simulink model "Sensor_actuator_test"  (R2020b)
settings: Solver=FixedStepAuto  StartTime=0.0  StopTime=inf  FixedStep=1  RelTol=1e-7  EnableMultiTasking=on
libraries: embdlinuxlib x12
settings Model: SimulationMode=external  Creator=enzlp  LastModifiedBy=Triphase_Setup
settings SolverCC: AlgebraicLoopSolver=LineSearch  PositivePriorityOrder=on
settings DataIOCC: SaveFormat=Array  ReturnWorkspaceOutputs=off
settings OptimizationCC: EnhancedBackFolding=on  PassReuseOutputArgsAs=Individual arguments  ZeroExternalMemoryAtStartup=off  ZeroInternalMemoryAtStartup=off  MaxStackSize=64  OptimizeBlockOrder=speed  DifferentSizesBufferReuse=on  OptimizationCustomize=off  EfficientTunableParamExpr=on
settings DebuggingCC: ParameterTunabilityLossMsg=error
settings HardwareCC: ProdBitPerPointer=32  ProdBitPerSizeT=32  ProdBitPerPtrDiffT=32  ProdLargestAtomicInteger=Long  ProdLargestAtomicFloat=Double  ProdWordSize=32  ProdLongLongMode=on  ProdHWDeviceType=ARM Compatible->ARM Cortex
settings RTWCC: Description=Embedded Coder  SystemTargetFile=ert.tlc  HardwareBoard=Raspberry Pi  TLCOptions="-aInlineSetEventsForThisBaseRateFcn=TLC_FALSE -aSuppressMultiTaskScheduler=TLC_FALSE  -aRateBasedStepFcn=0"  TemplateMakefile=ert_default_tmf  Toolchain=GNU GCC Raspberry Pi  BuildConfiguration=Faster Runs
settings CodeAppCC: ForceParamTrailComments=on  IgnoreCustomStorageClasses=off  OperatorAnnotations=on  SimulinkDataObjDesc=on  SFDataObjDesc=on  InsertBlockDesc=on
settings ERTTargetCC: TargetLangStandard=C99 (ISO)  SupportVariableSizeSignals=on  ExtMode=on  ExtModeTransport=2  ExtModeStaticAlloc=on  ExtModeMexFile=ext_xcp  ExtModeMexArgs='192.168.178.34' 0 17725  ExtModeIntrfLevel=Level2 - Open

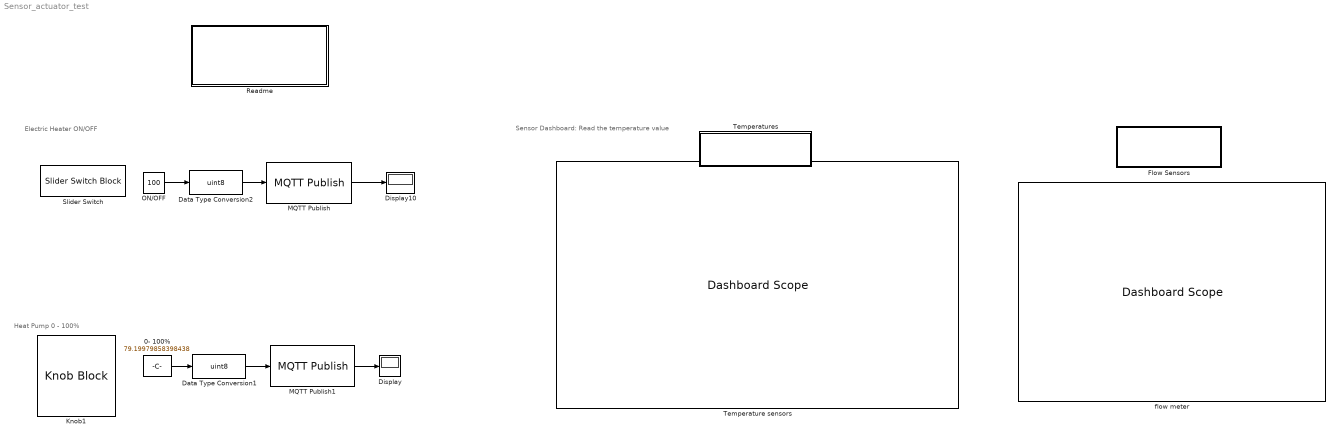
== system Sensor_actuator_test ==
  note: Heat Pump 0 - 100%
  note: Sensor Dashboard: Read the temperature value
  note: Electric Heater ON/OFF
  0- 100% : Constant  Value=79.19979858398438
  Data Type Conversion1 : DataTypeConversion  OutDataTypeStr=uint8
  Data Type Conversion2 : DataTypeConversion  OutDataTypeStr=uint8
  Display : Display
  Display10 : Display
  Flow Sensors : Subsystem
  Knob1 : KnobBlock
  MQTT Publish : embdlinuxlib/MQTT Publish  Topic=heatpump  QoS=0  RetainMsg=off
      settings: SourceProductBaseCode=SC_BEAGLEBONE_BLUE,NVIDIA,RASPPI
  MQTT Publish1 : embdlinuxlib/MQTT Publish  Topic=boiler  QoS=0  RetainMsg=off
      settings: SourceProductBaseCode=SC_BEAGLEBONE_BLUE,NVIDIA,RASPPI
  ON/OFF : Constant  Value=100
  Readme : Subsystem
  Slider Switch : SliderSwitchBlock
      settings: Values={{'Off', 'On'}, [0 1]}
  Temperature sensors : DashboardScope  Ymin=0  Ymax=30
  Temperatures : Subsystem
  flow meter : DashboardScope  Ymin=0  Ymax=30
  wires:
  0- 100%/1 -> Data Type Conversion1/1
  ON/OFF/1 -> Data Type Conversion2/1
  MQTT Publish1/1 -> Display/1
  MQTT Publish/1 -> Display10/1
  Data Type Conversion1/1 -> MQTT Publish1/1
  Data Type Conversion2/1 -> MQTT Publish/1

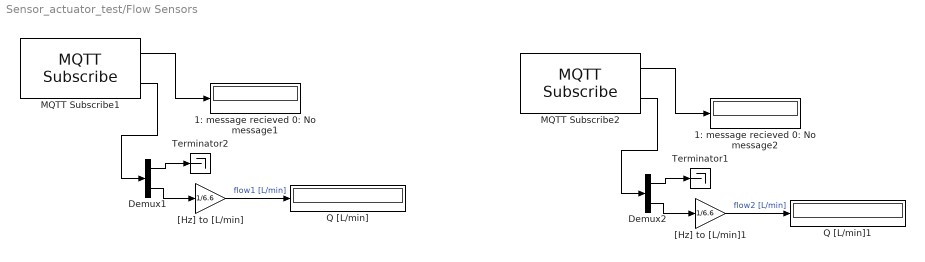
== system Sensor_actuator_test/Flow Sensors ==
  1: message recieved 0: No message1 : Display
  1: message recieved 0: No message2 : Display
  Demux1 : Demux  Outputs=2
  Demux2 : Demux  Outputs=2
  MQTT Subscribe1 : embdlinuxlib/MQTT Subscribe  Topic=flow1  QoS=0  MessageLength=2  SampleTime=1
      settings: SourceProductBaseCode=SC_BEAGLEBONE_BLUE,NVIDIA,RASPPI
  MQTT Subscribe2 : embdlinuxlib/MQTT Subscribe  Topic=flow2  QoS=0  MessageLength=2  SampleTime=1
      settings: SourceProductBaseCode=SC_BEAGLEBONE_BLUE,NVIDIA,RASPPI
  Q [L/min] : Display
  Q [L/min]1 : Display
  Terminator1 : Terminator
  Terminator2 : Terminator
  "[Hz] to [L/min]" : Gain  Gain=1/6.6
  "[Hz] to [L/min]1" : Gain  Gain=1/6.6
  wires:
  Demux1/1 -> Terminator2/1
  MQTT Subscribe1/1 -> 1: message recieved 0: No message1/1
  "[Hz] to [L/min]"/1 -> Q [L/min]/1  "flow1 [L/min]"
  MQTT Subscribe1/2 -> Demux1/1
  Demux1/2 -> "[Hz] to [L/min]"/1
  Demux2/2 -> "[Hz] to [L/min]1"/1
  "[Hz] to [L/min]1"/1 -> Q [L/min]1/1  "flow2 [L/min]"
  MQTT Subscribe2/2 -> Demux2/1
  MQTT Subscribe2/1 -> 1: message recieved 0: No message2/1
  Demux2/1 -> Terminator1/1

== system Sensor_actuator_test/Readme ==
  note: About :
      |
      | This Simulink file is used for testing the sensors and actuators connected to the OSEM hardware.
      |
      | There are two actuators in the system: The heat pump and the electric heater.
      |
      | There are four possible output ports in the OSEM board hardware, which can be addressed by the following names in the MQTT Publish block :
      |
      | - "Valve1": Analog output (0 - 100).
      | - "Valve2": Analog output (0 - 100).
      | - "Boiler": Analog output (0 - 100).
      | - "heatpump": Digital output (0 /1).
  note: Steps:
      |
      | Connect the hardware as described in the "about" section.
      |
      | In Simulink, under "Hardware tab", make sure the parameters of of the Raspberry PI are correct.
      |
      | Click "Monitor & Tune".
      |
      | The dashboard scopes should display the temperatures.
      |
      | By turning the knob and toggling the switch, test if the actuators reacts correctly to the setpoints.
      |
      | Use the knobs to change the setpoints of the heat pump and the electric heater. Verify on the hardware (Using a multimeter) that the physical signal corresponds to the setpoint.

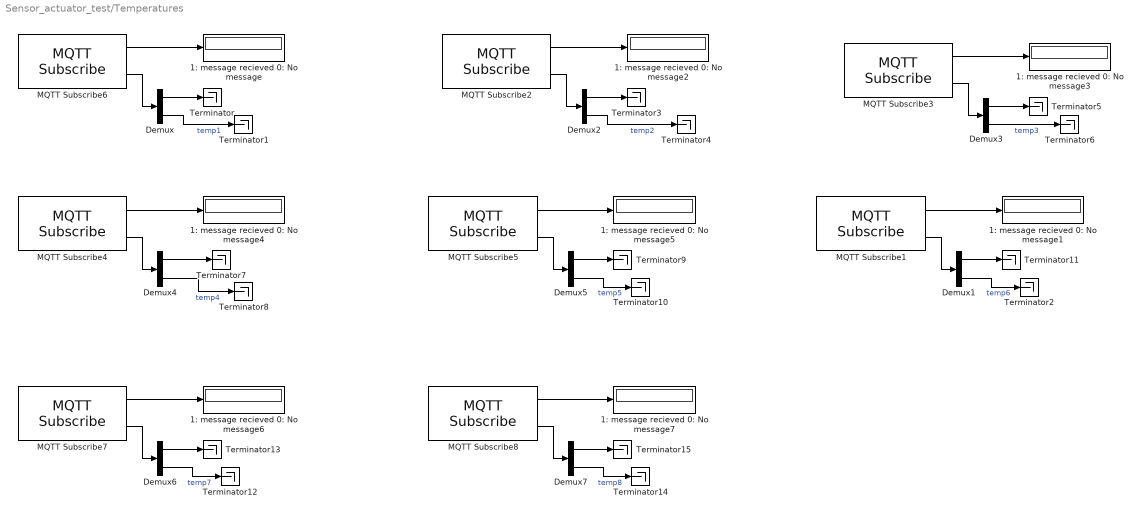
== system Sensor_actuator_test/Temperatures ==
  1: message recieved 0: No message{,1..7} (8 alike) : Display
  Demux{,1..7} (8 alike) : Demux  Outputs=2
  MQTT Subscribe1 : embdlinuxlib/MQTT Subscribe  Topic=temp6  QoS=0  MessageLength=2  SampleTime=1
      settings: SourceProductBaseCode=SC_BEAGLEBONE_BLUE,NVIDIA,RASPPI
  MQTT Subscribe2 : embdlinuxlib/MQTT Subscribe  Topic=temp2  QoS=0  MessageLength=2  SampleTime=1
      settings: SourceProductBaseCode=SC_BEAGLEBONE_BLUE,NVIDIA,RASPPI
  MQTT Subscribe3 : embdlinuxlib/MQTT Subscribe  Topic=temp3  QoS=0  MessageLength=2  SampleTime=1
      settings: SourceProductBaseCode=SC_BEAGLEBONE_BLUE,NVIDIA,RASPPI
  MQTT Subscribe4 : embdlinuxlib/MQTT Subscribe  Topic=temp4  QoS=0  MessageLength=2  SampleTime=1
      settings: SourceProductBaseCode=SC_BEAGLEBONE_BLUE,NVIDIA,RASPPI
  MQTT Subscribe5 : embdlinuxlib/MQTT Subscribe  Topic=temp5  QoS=0  MessageLength=2  SampleTime=1
      settings: SourceProductBaseCode=SC_BEAGLEBONE_BLUE,NVIDIA,RASPPI
  MQTT Subscribe6 : embdlinuxlib/MQTT Subscribe  Topic=temp1  QoS=0  MessageLength=2  SampleTime=1
      settings: SourceProductBaseCode=SC_BEAGLEBONE_BLUE,NVIDIA,RASPPI
  MQTT Subscribe7 : embdlinuxlib/MQTT Subscribe  Topic=temp7  QoS=0  MessageLength=2  SampleTime=1
      settings: SourceProductBaseCode=SC_BEAGLEBONE_BLUE,NVIDIA,RASPPI
  MQTT Subscribe8 : embdlinuxlib/MQTT Subscribe  Topic=temp8  QoS=0  MessageLength=2  SampleTime=1
      settings: SourceProductBaseCode=SC_BEAGLEBONE_BLUE,NVIDIA,RASPPI
  Terminator{,1..15} (16 alike) : Terminator
  wires:
  Demux/2 -> Terminator1/1  "temp1"
  MQTT Subscribe6/2 -> Demux/1
  MQTT Subscribe6/1 -> 1: message recieved 0: No message/1
  Demux2/1 -> Terminator3/1
  MQTT Subscribe4/1 -> 1: message recieved 0: No message4/1
  Demux3/2 -> Terminator6/1  "temp3"
  Demux4/1 -> Terminator7/1
  Demux3/1 -> Terminator5/1
  MQTT Subscribe3/1 -> 1: message recieved 0: No message3/1
  MQTT Subscribe2/2 -> Demux2/1
  Demux2/2 -> Terminator4/1  "temp2"
  Demux/1 -> Terminator/1
  Demux4/2 -> Terminator8/1  "temp4"
  Demux5/1 -> Terminator9/1
  MQTT Subscribe5/2 -> Demux5/1
  MQTT Subscribe3/2 -> Demux3/1
  Demux5/2 -> Terminator10/1  "temp5"
  MQTT Subscribe5/1 -> 1: message recieved 0: No message5/1
  MQTT Subscribe2/1 -> 1: message recieved 0: No message2/1
  MQTT Subscribe4/2 -> Demux4/1
  MQTT Subscribe1/1 -> 1: message recieved 0: No message1/1
  MQTT Subscribe1/2 -> Demux1/1
  Demux1/2 -> Terminator2/1  "temp6"
  Demux1/1 -> Terminator11/1
  MQTT Subscribe7/1 -> 1: message recieved 0: No message6/1
  MQTT Subscribe7/2 -> Demux6/1
  Demux6/2 -> Terminator12/1  "temp7"
  Demux6/1 -> Terminator13/1
  MQTT Subscribe8/1 -> 1: message recieved 0: No message7/1
  MQTT Subscribe8/2 -> Demux7/1
  Demux7/2 -> Terminator14/1  "temp8"
  Demux7/1 -> Terminator15/1
